simulink library "csc_swm_switch_state_model_collection_lib"  (R2014b)
settings: Solver=ode45  StartTime=0.0  StopTime=10.0  RelTol=1e-3
libraries: csu_swm_switch_state_model_lib x64, util_info_lib x1
settings Model: Creator=escrane  LastModifiedBy=mstewart

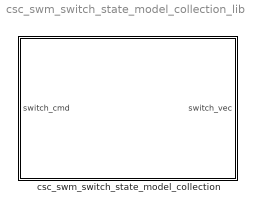
== system csc_swm_switch_state_model_collection_lib ==
  csc_swm_switch_state_model_collection : Subsystem
      mask Display: color('blue');text(0.05, 0.02, 'MoonEx', 'HorizontalAlignment', 'Left', 'VerticalAlignment', 'Bottom');color('red');text(0.95, 0.02, 'Autogenerated', 'HorizontalAlignment', 'Right', 'VerticalAlignment', 'Bottom');

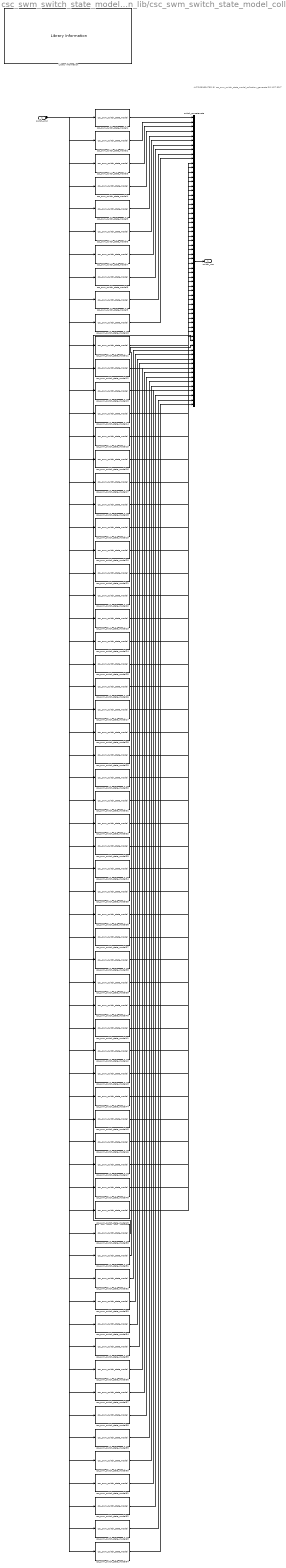
== system csc_swm_switch_state_model_collection_lib/csc_swm_switch_state_model_collection ==
  note: AUTOGENERATED BY csc_swm_switch_state_model_collection_generate
      | DO NOT EDIT
  switch_cmd : Inport
  Library Information : util_info_lib/Library Information  owner='NONE'
  csc_swm_switch_state_model1 : csu_swm_switch_state_model_lib/csu_swm_switch_state_model  switch_idx=1  num_switches=swm_num_switches
  csc_swm_switch_state_model10 : csu_swm_switch_state_model_lib/csu_swm_switch_state_model  switch_idx=10  num_switches=swm_num_switches
  csc_swm_switch_state_model11 : csu_swm_switch_state_model_lib/csu_swm_switch_state_model  switch_idx=11  num_switches=swm_num_switches
  csc_swm_switch_state_model12 : csu_swm_switch_state_model_lib/csu_swm_switch_state_model  switch_idx=12  num_switches=swm_num_switches
  csc_swm_switch_state_model13 : csu_swm_switch_state_model_lib/csu_swm_switch_state_model  switch_idx=13  num_switches=swm_num_switches
  csc_swm_switch_state_model14 : csu_swm_switch_state_model_lib/csu_swm_switch_state_model  switch_idx=14  num_switches=swm_num_switches
  csc_swm_switch_state_model15 : csu_swm_switch_state_model_lib/csu_swm_switch_state_model  switch_idx=15  num_switches=swm_num_switches
  csc_swm_switch_state_model16 : csu_swm_switch_state_model_lib/csu_swm_switch_state_model  switch_idx=16  num_switches=swm_num_switches
  csc_swm_switch_state_model17 : csu_swm_switch_state_model_lib/csu_swm_switch_state_model  switch_idx=17  num_switches=swm_num_switches
  csc_swm_switch_state_model18 : csu_swm_switch_state_model_lib/csu_swm_switch_state_model  switch_idx=18  num_switches=swm_num_switches
  csc_swm_switch_state_model19 : csu_swm_switch_state_model_lib/csu_swm_switch_state_model  switch_idx=19  num_switches=swm_num_switches
  csc_swm_switch_state_model2 : csu_swm_switch_state_model_lib/csu_swm_switch_state_model  switch_idx=2  num_switches=swm_num_switches
  csc_swm_switch_state_model20 : csu_swm_switch_state_model_lib/csu_swm_switch_state_model  switch_idx=20  num_switches=swm_num_switches
  csc_swm_switch_state_model21 : csu_swm_switch_state_model_lib/csu_swm_switch_state_model  switch_idx=21  num_switches=swm_num_switches
  csc_swm_switch_state_model22 : csu_swm_switch_state_model_lib/csu_swm_switch_state_model  switch_idx=22  num_switches=swm_num_switches
  csc_swm_switch_state_model23 : csu_swm_switch_state_model_lib/csu_swm_switch_state_model  switch_idx=23  num_switches=swm_num_switches
  csc_swm_switch_state_model24 : csu_swm_switch_state_model_lib/csu_swm_switch_state_model  switch_idx=24  num_switches=swm_num_switches
  csc_swm_switch_state_model25 : csu_swm_switch_state_model_lib/csu_swm_switch_state_model  switch_idx=25  num_switches=swm_num_switches
  csc_swm_switch_state_model26 : csu_swm_switch_state_model_lib/csu_swm_switch_state_model  switch_idx=26  num_switches=swm_num_switches
  csc_swm_switch_state_model27 : csu_swm_switch_state_model_lib/csu_swm_switch_state_model  switch_idx=27  num_switches=swm_num_switches
  csc_swm_switch_state_model28 : csu_swm_switch_state_model_lib/csu_swm_switch_state_model  switch_idx=28  num_switches=swm_num_switches
  csc_swm_switch_state_model29 : csu_swm_switch_state_model_lib/csu_swm_switch_state_model  switch_idx=29  num_switches=swm_num_switches
  csc_swm_switch_state_model3 : csu_swm_switch_state_model_lib/csu_swm_switch_state_model  switch_idx=3  num_switches=swm_num_switches
  csc_swm_switch_state_model30 : csu_swm_switch_state_model_lib/csu_swm_switch_state_model  switch_idx=30  num_switches=swm_num_switches
  csc_swm_switch_state_model31 : csu_swm_switch_state_model_lib/csu_swm_switch_state_model  switch_idx=31  num_switches=swm_num_switches
  csc_swm_switch_state_model32 : csu_swm_switch_state_model_lib/csu_swm_switch_state_model  switch_idx=32  num_switches=swm_num_switches
  csc_swm_switch_state_model33 : csu_swm_switch_state_model_lib/csu_swm_switch_state_model  switch_idx=33  num_switches=swm_num_switches
  csc_swm_switch_state_model34 : csu_swm_switch_state_model_lib/csu_swm_switch_state_model  switch_idx=34  num_switches=swm_num_switches
  csc_swm_switch_state_model35 : csu_swm_switch_state_model_lib/csu_swm_switch_state_model  switch_idx=35  num_switches=swm_num_switches
  csc_swm_switch_state_model36 : csu_swm_switch_state_model_lib/csu_swm_switch_state_model  switch_idx=36  num_switches=swm_num_switches
  csc_swm_switch_state_model37 : csu_swm_switch_state_model_lib/csu_swm_switch_state_model  switch_idx=37  num_switches=swm_num_switches
  csc_swm_switch_state_model38 : csu_swm_switch_state_model_lib/csu_swm_switch_state_model  switch_idx=38  num_switches=swm_num_switches
  csc_swm_switch_state_model39 : csu_swm_switch_state_model_lib/csu_swm_switch_state_model  switch_idx=39  num_switches=swm_num_switches
  csc_swm_switch_state_model4 : csu_swm_switch_state_model_lib/csu_swm_switch_state_model  switch_idx=4  num_switches=swm_num_switches
  csc_swm_switch_state_model40 : csu_swm_switch_state_model_lib/csu_swm_switch_state_model  switch_idx=40  num_switches=swm_num_switches
  csc_swm_switch_state_model41 : csu_swm_switch_state_model_lib/csu_swm_switch_state_model  switch_idx=41  num_switches=swm_num_switches
  csc_swm_switch_state_model42 : csu_swm_switch_state_model_lib/csu_swm_switch_state_model  switch_idx=42  num_switches=swm_num_switches
  csc_swm_switch_state_model43 : csu_swm_switch_state_model_lib/csu_swm_switch_state_model  switch_idx=43  num_switches=swm_num_switches
  csc_swm_switch_state_model44 : csu_swm_switch_state_model_lib/csu_swm_switch_state_model  switch_idx=44  num_switches=swm_num_switches
  csc_swm_switch_state_model45 : csu_swm_switch_state_model_lib/csu_swm_switch_state_model  switch_idx=45  num_switches=swm_num_switches
  csc_swm_switch_state_model46 : csu_swm_switch_state_model_lib/csu_swm_switch_state_model  switch_idx=46  num_switches=swm_num_switches
  csc_swm_switch_state_model47 : csu_swm_switch_state_model_lib/csu_swm_switch_state_model  switch_idx=47  num_switches=swm_num_switches
  csc_swm_switch_state_model48 : csu_swm_switch_state_model_lib/csu_swm_switch_state_model  switch_idx=48  num_switches=swm_num_switches
  csc_swm_switch_state_model49 : csu_swm_switch_state_model_lib/csu_swm_switch_state_model  switch_idx=49  num_switches=swm_num_switches
  csc_swm_switch_state_model5 : csu_swm_switch_state_model_lib/csu_swm_switch_state_model  switch_idx=5  num_switches=swm_num_switches
  csc_swm_switch_state_model50 : csu_swm_switch_state_model_lib/csu_swm_switch_state_model  switch_idx=50  num_switches=swm_num_switches
  csc_swm_switch_state_model51 : csu_swm_switch_state_model_lib/csu_swm_switch_state_model  switch_idx=51  num_switches=swm_num_switches
  csc_swm_switch_state_model52 : csu_swm_switch_state_model_lib/csu_swm_switch_state_model  switch_idx=52  num_switches=swm_num_switches
  csc_swm_switch_state_model53 : csu_swm_switch_state_model_lib/csu_swm_switch_state_model  switch_idx=53  num_switches=swm_num_switches
  csc_swm_switch_state_model54 : csu_swm_switch_state_model_lib/csu_swm_switch_state_model  switch_idx=54  num_switches=swm_num_switches
  csc_swm_switch_state_model55 : csu_swm_switch_state_model_lib/csu_swm_switch_state_model  switch_idx=55  num_switches=swm_num_switches
  csc_swm_switch_state_model56 : csu_swm_switch_state_model_lib/csu_swm_switch_state_model  switch_idx=56  num_switches=swm_num_switches
  csc_swm_switch_state_model57 : csu_swm_switch_state_model_lib/csu_swm_switch_state_model  switch_idx=57  num_switches=swm_num_switches
  csc_swm_switch_state_model58 : csu_swm_switch_state_model_lib/csu_swm_switch_state_model  switch_idx=58  num_switches=swm_num_switches
  csc_swm_switch_state_model59 : csu_swm_switch_state_model_lib/csu_swm_switch_state_model  switch_idx=59  num_switches=swm_num_switches
  csc_swm_switch_state_model6 : csu_swm_switch_state_model_lib/csu_swm_switch_state_model  switch_idx=6  num_switches=swm_num_switches
  csc_swm_switch_state_model60 : csu_swm_switch_state_model_lib/csu_swm_switch_state_model  switch_idx=60  num_switches=swm_num_switches
  csc_swm_switch_state_model61 : csu_swm_switch_state_model_lib/csu_swm_switch_state_model  switch_idx=61  num_switches=swm_num_switches
  csc_swm_switch_state_model62 : csu_swm_switch_state_model_lib/csu_swm_switch_state_model  switch_idx=62  num_switches=swm_num_switches
  csc_swm_switch_state_model63 : csu_swm_switch_state_model_lib/csu_swm_switch_state_model  switch_idx=63  num_switches=swm_num_switches
  csc_swm_switch_state_model64 : csu_swm_switch_state_model_lib/csu_swm_switch_state_model  switch_idx=64  num_switches=swm_num_switches
  csc_swm_switch_state_model7 : csu_swm_switch_state_model_lib/csu_swm_switch_state_model  switch_idx=7  num_switches=swm_num_switches
  csc_swm_switch_state_model8 : csu_swm_switch_state_model_lib/csu_swm_switch_state_model  switch_idx=8  num_switches=swm_num_switches
  csc_swm_switch_state_model9 : csu_swm_switch_state_model_lib/csu_swm_switch_state_model  switch_idx=9  num_switches=swm_num_switches
  switch_concatenate : Concatenate  NumInputs=64
  switch_vec : Outport
  wires:
  switch_concatenate/1 -> switch_vec/1
  switch_cmd/1 -> csc_swm_switch_state_model64/1, csc_swm_switch_state_model63/1, csc_swm_switch_state_model62/1, csc_swm_switch_state_model61/1, csc_swm_switch_state_model60/1, csc_swm_switch_state_model59/1, csc_swm_switch_state_model58/1, csc_swm_switch_state_model57/1, csc_swm_switch_state_model56/1, csc_swm_switch_state_model55/1, csc_swm_switch_state_model54/1, csc_swm_switch_state_model53/1, csc_swm_switch_state_model52/1, csc_swm_switch_state_model51/1, csc_swm_switch_state_model50/1, csc_swm_switch_state_model49/1, csc_swm_switch_state_model48/1, csc_swm_switch_state_model47/1, csc_swm_switch_state_model46/1, csc_swm_switch_state_model45/1, csc_swm_switch_state_model44/1, csc_swm_switch_state_model43/1, csc_swm_switch_state_model42/1, csc_swm_switch_state_model41/1, csc_swm_switch_state_model40/1, csc_swm_switch_state_model39/1, csc_swm_switch_state_model38/1, csc_swm_switch_state_model37/1, csc_swm_switch_state_model36/1, csc_swm_switch_state_model35/1, csc_swm_switch_state_model34/1, csc_swm_switch_state_model33/1, csc_swm_switch_state_model32/1, csc_swm_switch_state_model31/1, csc_swm_switch_state_model30/1, csc_swm_switch_state_model29/1, csc_swm_switch_state_model28/1, csc_swm_switch_state_model27/1, csc_swm_switch_state_model26/1, csc_swm_switch_state_model25/1, csc_swm_switch_state_model24/1, csc_swm_switch_state_model23/1, csc_swm_switch_state_model22/1, csc_swm_switch_state_model21/1, csc_swm_switch_state_model20/1, csc_swm_switch_state_model19/1, csc_swm_switch_state_model18/1, csc_swm_switch_state_model17/1, csc_swm_switch_state_model16/1, csc_swm_switch_state_model15/1, csc_swm_switch_state_model14/1, csc_swm_switch_state_model13/1, csc_swm_switch_state_model12/1, csc_swm_switch_state_model11/1, csc_swm_switch_state_model10/1, csc_swm_switch_state_model9/1, csc_swm_switch_state_model8/1, csc_swm_switch_state_model7/1, csc_swm_switch_state_model6/1, csc_swm_switch_state_model5/1, csc_swm_switch_state_model4/1, csc_swm_switch_state_model3/1, csc_swm_switch_state_model2/1, csc_swm_switch_state_model1/1
  csc_swm_switch_state_model64/1 -> switch_concatenate/64
  csc_swm_switch_state_model63/1 -> switch_concatenate/63
  csc_swm_switch_state_model62/1 -> switch_concatenate/62
  csc_swm_switch_state_model61/1 -> switch_concatenate/61
  csc_swm_switch_state_model60/1 -> switch_concatenate/60
  csc_swm_switch_state_model59/1 -> switch_concatenate/59
  csc_swm_switch_state_model58/1 -> switch_concatenate/58
  csc_swm_switch_state_model57/1 -> switch_concatenate/57
  csc_swm_switch_state_model56/1 -> switch_concatenate/56
  csc_swm_switch_state_model55/1 -> switch_concatenate/55
  csc_swm_switch_state_model54/1 -> switch_concatenate/54
  csc_swm_switch_state_model53/1 -> switch_concatenate/53
  csc_swm_switch_state_model52/1 -> switch_concatenate/52
  csc_swm_switch_state_model51/1 -> switch_concatenate/51
  csc_swm_switch_state_model50/1 -> switch_concatenate/50
  csc_swm_switch_state_model49/1 -> switch_concatenate/49
  csc_swm_switch_state_model48/1 -> switch_concatenate/48
  csc_swm_switch_state_model47/1 -> switch_concatenate/47
  csc_swm_switch_state_model46/1 -> switch_concatenate/46
  csc_swm_switch_state_model45/1 -> switch_concatenate/45
  csc_swm_switch_state_model44/1 -> switch_concatenate/44
  csc_swm_switch_state_model43/1 -> switch_concatenate/43
  csc_swm_switch_state_model42/1 -> switch_concatenate/42
  csc_swm_switch_state_model41/1 -> switch_concatenate/41
  csc_swm_switch_state_model40/1 -> switch_concatenate/40
  csc_swm_switch_state_model39/1 -> switch_concatenate/39
  csc_swm_switch_state_model38/1 -> switch_concatenate/38
  csc_swm_switch_state_model37/1 -> switch_concatenate/37
  csc_swm_switch_state_model36/1 -> switch_concatenate/36
  csc_swm_switch_state_model35/1 -> switch_concatenate/35
  csc_swm_switch_state_model34/1 -> switch_concatenate/34
  csc_swm_switch_state_model33/1 -> switch_concatenate/33
  csc_swm_switch_state_model32/1 -> switch_concatenate/32
  csc_swm_switch_state_model31/1 -> switch_concatenate/31
  csc_swm_switch_state_model30/1 -> switch_concatenate/30
  csc_swm_switch_state_model29/1 -> switch_concatenate/29
  csc_swm_switch_state_model28/1 -> switch_concatenate/28
  csc_swm_switch_state_model27/1 -> switch_concatenate/27
  csc_swm_switch_state_model26/1 -> switch_concatenate/26
  csc_swm_switch_state_model25/1 -> switch_concatenate/25
  csc_swm_switch_state_model24/1 -> switch_concatenate/24
  csc_swm_switch_state_model23/1 -> switch_concatenate/23
  csc_swm_switch_state_model22/1 -> switch_concatenate/22
  csc_swm_switch_state_model21/1 -> switch_concatenate/21
  csc_swm_switch_state_model20/1 -> switch_concatenate/20
  csc_swm_switch_state_model19/1 -> switch_concatenate/19
  csc_swm_switch_state_model18/1 -> switch_concatenate/18
  csc_swm_switch_state_model17/1 -> switch_concatenate/17
  csc_swm_switch_state_model16/1 -> switch_concatenate/16
  csc_swm_switch_state_model15/1 -> switch_concatenate/15
  csc_swm_switch_state_model14/1 -> switch_concatenate/14
  csc_swm_switch_state_model13/1 -> switch_concatenate/13
  csc_swm_switch_state_model12/1 -> switch_concatenate/12
  csc_swm_switch_state_model11/1 -> switch_concatenate/11
  csc_swm_switch_state_model10/1 -> switch_concatenate/10
  csc_swm_switch_state_model9/1 -> switch_concatenate/9
  csc_swm_switch_state_model8/1 -> switch_concatenate/8
  csc_swm_switch_state_model7/1 -> switch_concatenate/7
  csc_swm_switch_state_model6/1 -> switch_concatenate/6
  csc_swm_switch_state_model5/1 -> switch_concatenate/5
  csc_swm_switch_state_model4/1 -> switch_concatenate/4
  csc_swm_switch_state_model3/1 -> switch_concatenate/3
  csc_swm_switch_state_model2/1 -> switch_concatenate/2
  csc_swm_switch_state_model1/1 -> switch_concatenate/1
